simulink model "Motion_planner_Street_Drone"  (R2019b)
settings: Solver=FixedStepAuto  StartTime=0.0  StopTime=25  FixedStep=0.0075  MaxStep=1e-1  MinStep=1e-3  RelTol=1e-3  AbsTol=1e-4
InitFcn:
  | SD_init1
values from neighbouring files (symbols this model uses):
  cost = [2.71432892747 3.32441927977 3.79268757264 4.85642115368 6.12135035287 7.09825974303 9.57278659789 1.55754789407 1.51399555616 2.57723707661 3.8468529147 4.8336387623 ... (2430 elements, 1x2430)]    [matlab.mat]
  Front_brake = [0 2.2085352751 4.15209150797 6.12733711785 8.16604105928 9.79119154879 12.1808659635 14.1242630413 16.1155522836 18.1386900579 20.0839213981 22.1313006548 ... (68 elements, 34x2)]    [Front_brake.mat]
  N = size(X,1)    [curvature.m]
  obsx = [dx1 dx2 dx3 dx4]'    [dynamic_collison.m]    (also in dynamic_detection1.m = [x1 x2 x3 x4]')
  obsy = [dy1 dy2 dy3 dy4]'    [dynamic_collison.m]    (also in dynamic_detection1.m = [y1 y2 y3 y4]')
  x = obs_path(i,1)    [dynamic_collison.m]    (also in dynamic_detection1.m)
  X = [X]    [curvature.m]
  y = obs_path(i,2)    [dynamic_collison.m]    (also in dynamic_detection1.m)
undefined symbols (not defined in the file or in its folder): d, dfin, dini, Ki, Kp, L_0f, lookahead_time, lookahead_time_rev, Rear_brake, sigbuilder_block, steer_ratio, steer_sens, tfin, tini, TPS_0, xfin, Y, yfin, Z
libraries: sm_lib x290, nesl_utility x136, simulink x6, vrlib x2, powerlib_meascontrol x2
(part 3 of 14)

== system Motion_planner_Street_Drone/Trajectory Tracker/KM- StreetDrone/Street_Drone/Vehicle/FL_Suspension ==
  FL Cylinder : sm_lib/Body Elements/Revolved Solid  GraphicAmbientColor=[0.15 0.15 0.15 1.0]  BasedOnType=Mass  CenterOfMass=[0 0 0]  CenterOfMassUnits=m  GraphicDiffuseColor=[0.5 0.5 0.5]  Density=7850  DensityUnits=kg/(m^3)  DoExposeReferenceFrame=off  GraphicEmissiveColor=[0.0 0.0 0.0 1.0]  ExportEntireGeometry=off  SerializedFrames=<Frames><Frame><Id>Frame1</Id><Value><Name>F1</Name><Origin><Source>GeometricFeature</Source><FeatureName>side surface 1</FeatureName></Origin><PrimaryAxis><DefinedDirection>+Z</DefinedDirection><Source>ReferenceFrame</Source><SourceDirection>+Z</SourceDirection><FeatureName></FeatureName></PrimaryAxis><SecondaryAxis><DefinedDirection>+X</DefinedDirection><Source>ReferenceFrame</Source><SourceDirection>+X</SourceDirection><FeatureName></FeatureName></SecondaryAxis></Value></Frame></Frames>  MarkerShape=Sphere  MarkerSize=10  GraphicType=FromGeometry  InertiaType=CalculateFromGeometry  Mass=2  MassUnits=kg  MomentsOfInertia=[1 1 1]  MomentsOfInertiaUnits=kg*m^2  GraphicOpacity=0.6  ProductsOfInertia=[0 0 0]  ProductsOfInertiaUnits=kg*m^2  RevolutionCrossSection=cyl_xsec  RevolutionCrossSectionUnits=cm  RevolutionAngle=180  RevolutionAngleUnits=deg  RevolutionExtent=Full  GraphicShininess=75  GraphicSpecularColor=[0.5 0.5 0.5 1.0]  GraphicVisPropType=SimpleVisualProperties
  FL Piston : sm_lib/Body Elements/Revolved Solid  GraphicAmbientColor=[0.15 0.15 0.15 1.0]  BasedOnType=Mass  CenterOfMass=[0 0 0]  CenterOfMassUnits=m  GraphicDiffuseColor=[0.0 0.4 0.6]  Density=7850  DensityUnits=kg/(m^3)  DoExposeReferenceFrame=off  GraphicEmissiveColor=[0.0 0.0 0.0 1.0]  ExportEntireGeometry=off  SerializedFrames=<Frames><Frame><Id>Frame1</Id><Value><Name>F1</Name><Origin><Source>GeometricFeature</Source><FeatureName>side surface 3</FeatureName></Origin><PrimaryAxis><DefinedDirection>-Z</DefinedDirection><Source>ReferenceFrame</Source><SourceDirection>+Z</SourceDirection><FeatureName></FeatureName></PrimaryAxis><SecondaryAxis><DefinedDirection>+X</DefinedDirection><Source>ReferenceFrame</Source><SourceDirection>+X</SourceDirection><FeatureName></FeatureName></SecondaryAxis></Value></Frame><Frame><Id>Frame2</Id><Value><Name>F2</Name><Origin><Source>GeometricFeature</Source><FeatureName>side surface 1</FeatureName></Origin><PrimaryAxis><DefinedDirection>+Z</DefinedDirection><Source>ReferenceFrame</Source><SourceDirection>+Z</SourceDirection><FeatureName></FeatureName></PrimaryAxis><SecondaryAxis><DefinedDirection>+X</DefinedDirection><Source>ReferenceFrame</Source><SourceDirection>+X</SourceDirection><FeatureName></FeatureName></SecondaryAxis></Value></Frame></Frames>  MarkerShape=Sphere  MarkerSize=10  GraphicType=FromGeometry  InertiaType=CalculateFromGeometry  Mass=2  MassUnits=kg  MomentsOfInertia=[1 1 1]  MomentsOfInertiaUnits=kg*m^2  GraphicOpacity=1.0  ProductsOfInertia=[0 0 0]  ProductsOfInertiaUnits=kg*m^2  RevolutionCrossSection=piston_xsec  RevolutionCrossSectionUnits=cm  RevolutionAngle=180  RevolutionAngleUnits=deg  RevolutionExtent=Full  GraphicShininess=75  GraphicSpecularColor=[0.5 0.5 0.5 1.0]  GraphicVisPropType=SimpleVisualProperties
  PS-Simulink Converter{1..4,20} (5 alike) : nesl_utility/PS-Simulink Converter  PhysicalDomain=network_engine_domain  SubClassName=ps_output  LeftPortType=input  RightPortType=output  PseudoPeriodic=off  Frequencies=[]  Unit=inherit  AffineConversion=off
  Prismatic Joint1 : sm_lib/Joints/Prismatic Joint  JointMode=Normal  SenseConstraintForce=off  SenseConstraintForceX=off  SenseConstraintForceY=off  SenseConstraintForceZ=off  SenseConstraintTorque=off  SenseConstraintTorqueX=off  SenseConstraintTorqueY=off  SenseConstraintTorqueZ=off  SenseTotalForce=off  SenseTotalForceX=off  SenseTotalForceY=off  SenseTotalForceZ=off  SenseTotalTorque=off  SenseTotalTorqueX=off  SenseTotalTorqueY=off  SenseTotalTorqueZ=off  CompositeWrenchDir=FollowerOnBase  CompositeWrenchFrame=BaseFrame  EquilibriumPosition=0.1691  EquilibriumPositionUnits=m  SpringStiffness=50000  SpringStiffnessUnits=N/m  DampingCoefficient=3600  DampingCoefficientUnits=N/(m/s)  TorqueActuationMode=NoTorque  MotionActuationMode=ComputedMotion  SensePosition=on  SenseVelocity=on  SenseAcceleration=off  SenseTorqueForce=on  SenseLowerLimitTorqueForce=on  SenseUpperLimitTorqueForce=on  LowerLimitSpecify=off  LowerLimitBound=0.1  LowerLimitBoundUnits=m  LowerLimitStiffness=60000  LowerLimitStiffnessUnits=N/m  LowerLimitDamping=2000  LowerLimitDampingUnits=N/(m/s)  LowerLimitTransitionRegionWidth=1e-4  LowerLimitTransitionRegionWidthUnits=m  UpperLimitSpecify=off  UpperLimitBound=0.16  UpperLimitBoundUnits=m  UpperLimitStiffness=283333.33  UpperLimitStiffnessUnits=N/m  UpperLimitDamping=2000  UpperLimitDampingUnits=N/(m/s)  UpperLimitTransitionRegionWidth=1e-4  UpperLimitTransitionRegionWidthUnits=m  PositionTargetSpecify=on  PositionTargetPriority=High  PositionTargetValue=0.1691  PositionTargetValueUnits=m  VelocityTargetSpecify=off  VelocityTargetPriority=High  VelocityTargetValue=0  VelocityTargetValueUnits=m/s
  Rigid Transform : sm_lib/Frames and Transforms/Rigid Transform  TranslationMethod=Cartesian  TranslationStandardOffset=0  TranslationLengthUnit=m  TranslationStandardAxis=+Z  TranslationCartesianOffset=[0.90996 0.32189 0.16271]  TranslationROffset=0  TranslationROffsetUnits=m  TranslationZOffset=0  TranslationZOffsetUnits=m  TranslationThetaOffset=0  TranslationThetaOffsetUnits=deg  RotationMethod=None  RotationAngleUnits=deg  RotationStandardAxis=+Z  RotationAngle=0.0  RotationArbitraryAxis=[0 0 1]  FollAlignAxisA=+X  BaseAlignAxisA=+Y  FollAlignAxisB=+Y  BaseAlignAxisB=+Z  RotationSequenceAxes=FollowerAxes  RotationSequence=XYX  RotationSequenceAngles=[0 0 0]  RotationSequenceAnglesUnits=deg  RotationMatrix=[1 0 0; 0 1 0; 0 0 1]
  Rigid Transform2 : sm_lib/Frames and Transforms/Rigid Transform  TranslationMethod=None  TranslationStandardOffset=0  TranslationLengthUnit=m  TranslationStandardAxis=+Z  TranslationCartesianOffset=[0 0 0]  TranslationROffset=0  TranslationROffsetUnits=m  TranslationZOffset=0  TranslationZOffsetUnits=m  TranslationThetaOffset=0  TranslationThetaOffsetUnits=deg  RotationMethod=StandardAxis  RotationAngleUnits=deg  RotationStandardAxis=+Z  RotationAngle=24.85  RotationArbitraryAxis=[0 0 1]  FollAlignAxisA=+X  BaseAlignAxisA=+Y  FollAlignAxisB=+Y  BaseAlignAxisB=+Z  RotationSequenceAxes=FollowerAxes  RotationSequence=XYX  RotationSequenceAngles=[0 0 0]  RotationSequenceAnglesUnits=deg  RotationMatrix=[1 0 0; 0 1 0; 0 0 1]
  Rigid Transform55 : sm_lib/Frames and Transforms/Rigid Transform  TranslationMethod=None  TranslationStandardOffset=0  TranslationLengthUnit=m  TranslationStandardAxis=+Z  TranslationCartesianOffset=[0.90996 0.32189 0.16271]  TranslationROffset=0  TranslationROffsetUnits=m  TranslationZOffset=0  TranslationZOffsetUnits=m  TranslationThetaOffset=0  TranslationThetaOffsetUnits=deg  RotationMethod=StandardAxis  RotationAngleUnits=deg  RotationStandardAxis=+X  RotationAngle=180  RotationArbitraryAxis=[0 0 1]  FollAlignAxisA=+X  BaseAlignAxisA=+Y  FollAlignAxisB=+Y  BaseAlignAxisB=+Z  RotationSequenceAxes=FollowerAxes  RotationSequence=XYX  RotationSequenceAngles=[0 0 0]  RotationSequenceAnglesUnits=deg  RotationMatrix=[1 0 0; 0 1 0; 0 0 1]
  Scope1 : Scope
  Scope2 : Scope
  Scope9 : Scope  NumInputPorts=3
  Spherical Joint : sm_lib/Joints/Spherical Joint  JointMode=Normal  SenseConstraintForce=off  SenseConstraintForceX=off  SenseConstraintForceY=off  SenseConstraintForceZ=off  SenseConstraintTorque=off  SenseConstraintTorqueX=off  SenseConstraintTorqueY=off  SenseConstraintTorqueZ=off  SenseTotalForce=off  SenseTotalForceX=off  SenseTotalForceY=off  SenseTotalForceZ=off  SenseTotalTorque=off  SenseTotalTorqueX=off  SenseTotalTorqueY=off  SenseTotalTorqueZ=off  CompositeWrenchDir=FollowerOnBase  CompositeWrenchFrame=BaseFrame  DefPosRotationMethod=None  DefPosRotationAngleUnits=deg  DefPosRotationStandardAxis=+Z  DefPosRotationAngle=0.0  DefPosRotationArbitraryAxis=[0 0 1]  DefPosFollAlignAxisA=+X  DefPosBaseAlignAxisA=+Y  DefPosFollAlignAxisB=+Y  DefPosBaseAlignAxisB=+Z  DefPosRotationSequenceAxes=FollowerAxes  DefPosRotationSequence=XYX  DefPosRotationSequenceAngles=[0 0 0]  DefPosRotationSequenceAnglesUnits=deg  DefPosRotationMatrix=[1 0 0; 0 1 0; 0 0 1]  EqPosRotationMethod=None  EqPosRotationAngleUnits=deg  EqPosRotationStandardAxis=+Z  EqPosRotationAngle=0.0  EqPosRotationArbitraryAxis=[0 0 1]  EqPosFollAlignAxisA=+X  EqPosBaseAlignAxisA=+Y  EqPosFollAlignAxisB=+Y  EqPosBaseAlignAxisB=+Z  EqPosRotationSequenceAxes=FollowerAxes  EqPosRotationSequence=XYX  EqPosRotationSequenceAngles=[0 0 0]  EqPosRotationSequenceAnglesUnits=deg  EqPosRotationMatrix=[1 0 0; 0 1 0; 0 0 1]  SpringStiffness=0  SpringStiffnessUnits=N*m/deg  DampingCoefficient=0  DampingCoefficientUnits=N*m/(deg/s)  ActuateTorqueX=on  ActuateTorqueY=on  ActuateTorqueZ=on  ActuateTorque=off  TorqueActuationMode=NoTorque  MotionActuationMode=ComputedMotion  ActuationFrame=BaseFrame  SensePosition=off  SenseVelocityX=off  SenseVelocityY=off  SenseVelocityZ=off  SenseVelocity=off  SenseAccelerationX=off  SenseAccelerationY=off  SenseAccelerationZ=off  SenseAcceleration=off  SenseTorqueX=off  SenseTorqueY=off  SenseTorqueZ=off  SenseTorqueForce=off  SenseLowerLimitTorqueMag=off  SenseUpperLimitTorqueMag=off  SensingFrame=BaseFrame  LowerLimitSpecify=off  LowerLimitBound=15  LowerLimitBoundUnits=deg  LowerLimitStiffness=1e4  LowerLimitStiffnessUnits=N*m/deg  LowerLimitDamping=10  LowerLimitDampingUnits=N*m/(deg/s)  LowerLimitTransitionRegionWidth=0.1  LowerLimitTransitionRegionWidthUnits=deg  UpperLimitSpecify=off  UpperLimitBound=45  UpperLimitBoundUnits=deg  UpperLimitStiffness=1e4  UpperLimitStiffnessUnits=N*m/deg  UpperLimitDamping=10  UpperLimitDampingUnits=N*m/(deg/s)  UpperLimitTransitionRegionWidth=0.1  UpperLimitTransitionRegionWidthUnits=deg  PositionTargetRotationMethod=None  PositionTargetRotationAngleUnits=deg  PositionTargetRotationStandardAxis=+Z  PositionTargetRotationAngle=0.0  PositionTargetRotationArbitraryAxis=[0 0 1]  PositionTargetFollAlignAxisA=+X  PositionTargetBaseAlignAxisA=+Y  PositionTargetFollAlignAxisB=+Y  PositionTargetBaseAlignAxisB=+Z  PositionTargetRotationSequenceAxes=FollowerAxes  PositionTargetRotationSequence=XYX  PositionTargetRotationSequenceAngles=[0 0 0]  PositionTargetRotationSequenceAnglesUnits=deg  PositionTargetRotationMatrix=[1 0 0; 0 1 0; 0 0 1]  PositionTargetSpecify=off  PositionTargetPriority=High  VelocityTargetValue=[0 0 0]  VelocityTargetValueUnits=deg/s  VelocityTargetSpecify=off  VelocityTargetPriority=Low  VelocityTargetInFollowerFrame=off
  steering_angle_measurement : Subsystem
  chassis : PMIOPort  Side=Left
  upright : PMIOPort  Port=2  Side=Right
  wires:
  PS-Simulink Converter4/1 -> Scope9/3
  PS-Simulink Converter3/1 -> Scope9/2
  PS-Simulink Converter2/1 -> Scope9/1
  PS-Simulink Converter1/1 -> Scope2/1
  PS-Simulink Converter20/1 -> Scope1/1
  connections:
  Prismatic Joint1/RConn6 -- PS-Simulink Converter4/LConn1
  Prismatic Joint1/RConn5 -- PS-Simulink Converter3/LConn1
  Prismatic Joint1/RConn4 -- PS-Simulink Converter2/LConn1
  Prismatic Joint1/RConn3 -- PS-Simulink Converter1/LConn1
  Rigid Transform2/RConn1 -- upright/RConn1
  Prismatic Joint1/LConn1 -- FL Cylinder/LConn1 -- steering_angle_measurement/RConn1 -- Rigid Transform55/RConn1
  steering_angle_measurement/LConn1 -- chassis/RConn1 -- Rigid Transform/LConn1
  Spherical Joint/LConn1 -- Rigid Transform/RConn1
  Spherical Joint/RConn1 -- Rigid Transform55/LConn1
  FL Piston/RConn1 -- Rigid Transform2/LConn1
  Prismatic Joint1/RConn1 -- FL Piston/LConn1
  Prismatic Joint1/RConn2 -- PS-Simulink Converter20/LConn1

== system Motion_planner_Street_Drone/Trajectory Tracker/KM- StreetDrone/Street_Drone/Vehicle/FL_Upright ==
  Cylindrical Solid1 : sm_lib/Body Elements/Cylindrical Solid  GraphicAmbientColor=[0.15 0.15 0.15 1.0]  BasedOnType=Mass  CenterOfMass=[0 0 0]  CenterOfMassUnits=m  GraphicDiffuseColor=[0.5 0.5 0.5]  CylinderLength=19.061  CylinderLengthUnits=cm  CylinderRadius=1  CylinderRadiusUnits=cm  Density=1000  DensityUnits=kg/m^3  DoExposeReferenceFrame=off  GraphicEmissiveColor=[0.0 0.0 0.0 1.0]  ExportEntireGeometry=off  SerializedFrames=<Frames><Frame><Id>Frame1</Id><Value><Name>F1</Name><Origin><Source>GeometricFeature</Source><FeatureName>top surface</FeatureName></Origin><PrimaryAxis><DefinedDirection>+Z</DefinedDirection><Source>ReferenceFrame</Source><SourceDirection>+Z</SourceDirection><FeatureName></FeatureName></PrimaryAxis><SecondaryAxis><DefinedDirection>+X</DefinedDirection><Source>ReferenceFrame</Source><SourceDirection>+X</SourceDirection><FeatureName></FeatureName></SecondaryAxis></Value></Frame><Frame><Id>Frame2</Id><Value><Name>F2</Name><Origin><Source>GeometricFeature</Source><FeatureName>bottom surface</FeatureName></Origin><PrimaryAxis><DefinedDirection>+Z</DefinedDirection><Source>ReferenceFrame</Source><SourceDirection>+Z</SourceDirection><FeatureName></FeatureName></PrimaryAxis><SecondaryAxis><DefinedDirection>+X</DefinedDirection><Source>ReferenceFrame</Source><SourceDirection>+X</SourceDirection><FeatureName></FeatureName></SecondaryAxis></Value></Frame></Frames>  MarkerShape=Sphere  MarkerSize=10  GraphicType=FromGeometry  InertiaType=CalculateFromGeometry  Mass=3.5  MassUnits=kg  MomentsOfInertia=[0.0001 0.0001 0.0001]  MomentsOfInertiaUnits=kg*m^2  GraphicOpacity=1.0  ProductsOfInertia=[0 0 0]  ProductsOfInertiaUnits=kg*m^2  GraphicShininess=75  GraphicSpecularColor=[0.5 0.5 0.5 1.0]  GraphicVisPropType=SimpleVisualProperties
  Cylindrical Solid10 : sm_lib/Body Elements/Cylindrical Solid  GraphicAmbientColor=[0.15 0.15 0.15 1.0]  BasedOnType=Density  CenterOfMass=[0 0 0]  CenterOfMassUnits=m  GraphicDiffuseColor=[0.5 0.5 0.5]  CylinderLength=4.72  CylinderLengthUnits=cm  CylinderRadius=1  CylinderRadiusUnits=cm  Density=1000  DensityUnits=kg/m^3  DoExposeReferenceFrame=off  GraphicEmissiveColor=[0.0 0.0 0.0 1.0]  ExportEntireGeometry=off  SerializedFrames=<Frames><Frame><Id>Frame1</Id><Value><Name>F1</Name><Origin><Source>GeometricFeature</Source><FeatureName>top surface</FeatureName></Origin><PrimaryAxis><DefinedDirection>+Z</DefinedDirection><Source>ReferenceFrame</Source><SourceDirection>+Z</SourceDirection><FeatureName></FeatureName></PrimaryAxis><SecondaryAxis><DefinedDirection>+X</DefinedDirection><Source>ReferenceFrame</Source><SourceDirection>+X</SourceDirection><FeatureName></FeatureName></SecondaryAxis></Value></Frame><Frame><Id>Frame2</Id><Value><Name>F2</Name><Origin><Source>GeometricFeature</Source><FeatureName>bottom surface</FeatureName></Origin><PrimaryAxis><DefinedDirection>+Z</DefinedDirection><Source>ReferenceFrame</Source><SourceDirection>+Z</SourceDirection><FeatureName></FeatureName></PrimaryAxis><SecondaryAxis><DefinedDirection>+X</DefinedDirection><Source>ReferenceFrame</Source><SourceDirection>+X</SourceDirection><FeatureName></FeatureName></SecondaryAxis></Value></Frame></Frames>  MarkerShape=Sphere  MarkerSize=10  GraphicType=FromGeometry  InertiaType=Custom  Mass=0  MassUnits=kg  MomentsOfInertia=[0 0 0]  MomentsOfInertiaUnits=kg*m^2  GraphicOpacity=1.0  ProductsOfInertia=[0 0 0]  ProductsOfInertiaUnits=kg*m^2  GraphicShininess=75  GraphicSpecularColor=[0.5 0.5 0.5 1.0]  GraphicVisPropType=SimpleVisualProperties
  Cylindrical Solid2 : sm_lib/Body Elements/Cylindrical Solid  GraphicAmbientColor=[0.15 0.15 0.15 1.0]  BasedOnType=Density  CenterOfMass=[0 0 0]  CenterOfMassUnits=m  GraphicDiffuseColor=[0.5 0.5 0.5]  CylinderLength=5  CylinderLengthUnits=cm  CylinderRadius=1  CylinderRadiusUnits=cm  Density=1000  DensityUnits=kg/m^3  DoExposeReferenceFrame=off  GraphicEmissiveColor=[0.0 0.0 0.0 1.0]  ExportEntireGeometry=off  SerializedFrames=<Frames><Frame><Id>Frame1</Id><Value><Name>F1</Name><Origin><Source>GeometricFeature</Source><FeatureName>top surface</FeatureName></Origin><PrimaryAxis><DefinedDirection>+Z</DefinedDirection><Source>ReferenceFrame</Source><SourceDirection>+Z</SourceDirection><FeatureName></FeatureName></PrimaryAxis><SecondaryAxis><DefinedDirection>+X</DefinedDirection><Source>ReferenceFrame</Source><SourceDirection>+X</SourceDirection><FeatureName></FeatureName></SecondaryAxis></Value></Frame><Frame><Id>Frame2</Id><Value><Name>F2</Name><Origin><Source>GeometricFeature</Source><FeatureName>bottom surface</FeatureName></Origin><PrimaryAxis><DefinedDirection>+Z</DefinedDirection><Source>ReferenceFrame</Source><SourceDirection>+Z</SourceDirection><FeatureName></FeatureName></PrimaryAxis><SecondaryAxis><DefinedDirection>+X</DefinedDirection><Source>ReferenceFrame</Source><SourceDirection>+X</SourceDirection><FeatureName></FeatureName></SecondaryAxis></Value></Frame></Frames>  MarkerShape=Sphere  MarkerSize=10  GraphicType=FromGeometry  InertiaType=Custom  Mass=0  MassUnits=kg  MomentsOfInertia=[0 0 0]  MomentsOfInertiaUnits=kg*m^2  GraphicOpacity=1.0  ProductsOfInertia=[0 0 0]  ProductsOfInertiaUnits=kg*m^2  GraphicShininess=75  GraphicSpecularColor=[0.5 0.5 0.5 1.0]  GraphicVisPropType=SimpleVisualProperties
  Cylindrical Solid9 : sm_lib/Body Elements/Cylindrical Solid  GraphicAmbientColor=[0.15 0.15 0.15 1.0]  BasedOnType=Density  CenterOfMass=[0 0 0]  CenterOfMassUnits=m  GraphicDiffuseColor=[0.5 0.5 0.5]  CylinderLength=7.9  CylinderLengthUnits=cm  CylinderRadius=1  CylinderRadiusUnits=cm  Density=1000  DensityUnits=kg/m^3  DoExposeReferenceFrame=off  GraphicEmissiveColor=[0.0 0.0 0.0 1.0]  ExportEntireGeometry=off  SerializedFrames=<Frames><Frame><Id>Frame1</Id><Value><Name>F1</Name><Origin><Source>GeometricFeature</Source><FeatureName>top surface</FeatureName></Origin><PrimaryAxis><DefinedDirection>+Z</DefinedDirection><Source>ReferenceFrame</Source><SourceDirection>+Z</SourceDirection><FeatureName></FeatureName></PrimaryAxis><SecondaryAxis><DefinedDirection>+X</DefinedDirection><Source>ReferenceFrame</Source><SourceDirection>+X</SourceDirection><FeatureName></FeatureName></SecondaryAxis></Value></Frame><Frame><Id>Frame2</Id><Value><Name>F2</Name><Origin><Source>GeometricFeature</Source><FeatureName>bottom surface</FeatureName></Origin><PrimaryAxis><DefinedDirection>+Z</DefinedDirection><Source>ReferenceFrame</Source><SourceDirection>+Z</SourceDirection><FeatureName></FeatureName></PrimaryAxis><SecondaryAxis><DefinedDirection>+X</DefinedDirection><Source>ReferenceFrame</Source><SourceDirection>+X</SourceDirection><FeatureName></FeatureName></SecondaryAxis></Value></Frame></Frames>  MarkerShape=Sphere  MarkerSize=10  GraphicType=FromGeometry  InertiaType=Custom  Mass=0  MassUnits=kg  MomentsOfInertia=[0 0 0]  MomentsOfInertiaUnits=kg*m^2  GraphicOpacity=1.0  ProductsOfInertia=[0 0 0]  ProductsOfInertiaUnits=kg*m^2  GraphicShininess=75  GraphicSpecularColor=[0.5 0.5 0.5 1.0]  GraphicVisPropType=SimpleVisualProperties
  Rigid Transform11 : sm_lib/Frames and Transforms/Rigid Transform  TranslationMethod=StandardAxis  TranslationStandardOffset=9.929  TranslationLengthUnit=cm  TranslationStandardAxis=+Z  TranslationCartesianOffset=[0 0 0]  TranslationROffset=0  TranslationROffsetUnits=m  TranslationZOffset=0  TranslationZOffsetUnits=m  TranslationThetaOffset=0  TranslationThetaOffsetUnits=deg  RotationMethod=StandardAxis  RotationAngleUnits=deg  RotationStandardAxis=+X  RotationAngle=90  RotationArbitraryAxis=[0 0 1]  FollAlignAxisA=+X  BaseAlignAxisA=+Y  FollAlignAxisB=+Y  BaseAlignAxisB=+Z  RotationSequenceAxes=FollowerAxes  RotationSequence=XYX  RotationSequenceAngles=[0 0 0]  RotationSequenceAnglesUnits=deg  RotationMatrix=[1 0 0; 0 1 0; 0 0 1]
  Rigid Transform12 : sm_lib/Frames and Transforms/Rigid Transform  TranslationMethod=StandardAxis  TranslationStandardOffset=0.5  TranslationLengthUnit=cm  TranslationStandardAxis=+Y  TranslationCartesianOffset=[0 0 0]  TranslationROffset=0  TranslationROffsetUnits=m  TranslationZOffset=0  TranslationZOffsetUnits=m  TranslationThetaOffset=0  TranslationThetaOffsetUnits=deg  RotationMethod=StandardAxis  RotationAngleUnits=deg  RotationStandardAxis=-X  RotationAngle=89  RotationArbitraryAxis=[0 0 1]  FollAlignAxisA=+X  BaseAlignAxisA=+Y  FollAlignAxisB=+Y  BaseAlignAxisB=+Z  RotationSequenceAxes=FollowerAxes  RotationSequence=XYX  RotationSequenceAngles=[0 0 0]  RotationSequenceAnglesUnits=deg  RotationMatrix=[1 0 0; 0 1 0; 0 0 1]
  Rigid Transform14 : sm_lib/Frames and Transforms/Rigid Transform  TranslationMethod=StandardAxis  TranslationStandardOffset=0.5  TranslationLengthUnit=cm  TranslationStandardAxis=-Y  TranslationCartesianOffset=[0 0 0]  TranslationROffset=0  TranslationROffsetUnits=m  TranslationZOffset=0  TranslationZOffsetUnits=m  TranslationThetaOffset=0  TranslationThetaOffsetUnits=deg  RotationMethod=StandardAxis  RotationAngleUnits=deg  RotationStandardAxis=-X  RotationAngle=88  RotationArbitraryAxis=[0 0 1]  FollAlignAxisA=+X  BaseAlignAxisA=+Y  FollAlignAxisB=+Y  BaseAlignAxisB=+Z  RotationSequenceAxes=FollowerAxes  RotationSequence=XYX  RotationSequenceAngles=[0 0 0]  RotationSequenceAnglesUnits=deg  RotationMatrix=[1 0 0; 0 1 0; 0 0 1]
  Rigid Transform15 : sm_lib/Frames and Transforms/Rigid Transform  TranslationMethod=None  TranslationStandardOffset=0  TranslationLengthUnit=m  TranslationStandardAxis=+Z  TranslationCartesianOffset=[0 0 0]  TranslationROffset=0  TranslationROffsetUnits=m  TranslationZOffset=0  TranslationZOffsetUnits=m  TranslationThetaOffset=0  TranslationThetaOffsetUnits=deg  RotationMethod=StandardAxis  RotationAngleUnits=deg  RotationStandardAxis=+Y  RotationAngle=180  RotationArbitraryAxis=[0 0 1]  FollAlignAxisA=+X  BaseAlignAxisA=+Y  FollAlignAxisB=+Y  BaseAlignAxisB=+Z  RotationSequenceAxes=FollowerAxes  RotationSequence=XYX  RotationSequenceAngles=[0 0 0]  RotationSequenceAnglesUnits=deg  RotationMatrix=[1 0 0; 0 1 0; 0 0 1]
  Rigid Transform16 : sm_lib/Frames and Transforms/Rigid Transform  TranslationMethod=None  TranslationStandardOffset=9.132  TranslationLengthUnit=cm  TranslationStandardAxis=-Z  TranslationCartesianOffset=[0 0 0]  TranslationROffset=0  TranslationROffsetUnits=m  TranslationZOffset=0  TranslationZOffsetUnits=m  TranslationThetaOffset=0  TranslationThetaOffsetUnits=deg  RotationMethod=StandardAxis  RotationAngleUnits=deg  RotationStandardAxis=+X  RotationAngle=-73  RotationArbitraryAxis=[0 0 1]  FollAlignAxisA=+X  BaseAlignAxisA=+Y  FollAlignAxisB=+Y  BaseAlignAxisB=+Z  RotationSequenceAxes=FollowerAxes  RotationSequence=XYX  RotationSequenceAngles=[0 0 0]  RotationSequenceAnglesUnits=deg  RotationMatrix=[1 0 0; 0 1 0; 0 0 1]
  Rigid Transform17 : sm_lib/Frames and Transforms/Rigid Transform  TranslationMethod=None  TranslationStandardOffset=9.132  TranslationLengthUnit=cm  TranslationStandardAxis=-Z  TranslationCartesianOffset=[0 0 0]  TranslationROffset=0  TranslationROffsetUnits=m  TranslationZOffset=0  TranslationZOffsetUnits=m  TranslationThetaOffset=0  TranslationThetaOffsetUnits=deg  RotationMethod=StandardAxis  RotationAngleUnits=deg  RotationStandardAxis=+X  RotationAngle=-90  RotationArbitraryAxis=[0 0 1]  FollAlignAxisA=+X  BaseAlignAxisA=+Y  FollAlignAxisB=+Y  BaseAlignAxisB=+Z  RotationSequenceAxes=FollowerAxes  RotationSequence=XYX  RotationSequenceAngles=[0 0 0]  RotationSequenceAnglesUnits=deg  RotationMatrix=[1 0 0; 0 1 0; 0 0 1]
  Rigid Transform56 : sm_lib/Frames and Transforms/Rigid Transform  TranslationMethod=StandardAxis  TranslationStandardOffset=9.929  TranslationLengthUnit=cm  TranslationStandardAxis=+Z  TranslationCartesianOffset=[0 0 0]  TranslationROffset=0  TranslationROffsetUnits=m  TranslationZOffset=0  TranslationZOffsetUnits=m  TranslationThetaOffset=0  TranslationThetaOffsetUnits=deg  RotationMethod=StandardAxis  RotationAngleUnits=deg  RotationStandardAxis=-Y  RotationAngle=98.5  RotationArbitraryAxis=[0 0 1]  FollAlignAxisA=+X  BaseAlignAxisA=+Y  FollAlignAxisB=+Y  BaseAlignAxisB=+Z  RotationSequenceAxes=FollowerAxes  RotationSequence=XYX  RotationSequenceAngles=[0 0 0]  RotationSequenceAnglesUnits=deg  RotationMatrix=[1 0 0; 0 1 0; 0 0 1]
  Rigid Transform60 : sm_lib/Frames and Transforms/Rigid Transform  TranslationMethod=None  TranslationStandardOffset=9.929  TranslationLengthUnit=cm  TranslationStandardAxis=+Z  TranslationCartesianOffset=[0 0 0]  TranslationROffset=0  TranslationROffsetUnits=m  TranslationZOffset=0  TranslationZOffsetUnits=m  TranslationThetaOffset=0  TranslationThetaOffsetUnits=deg  RotationMethod=StandardAxis  RotationAngleUnits=deg  RotationStandardAxis=-X  RotationAngle=90  RotationArbitraryAxis=[0 0 1]  FollAlignAxisA=+X  BaseAlignAxisA=+Y  FollAlignAxisB=+Y  BaseAlignAxisB=+Z  RotationSequenceAxes=FollowerAxes  RotationSequence=XYX  RotationSequenceAngles=[0 0 0]  RotationSequenceAnglesUnits=deg  RotationMatrix=[1 0 0; 0 1 0; 0 0 1]
  Rigid Transform61 : sm_lib/Frames and Transforms/Rigid Transform  TranslationMethod=None  TranslationStandardOffset=9.929  TranslationLengthUnit=cm  TranslationStandardAxis=+Z  TranslationCartesianOffset=[0 0 0]  TranslationROffset=0  TranslationROffsetUnits=m  TranslationZOffset=0  TranslationZOffsetUnits=m  TranslationThetaOffset=0  TranslationThetaOffsetUnits=deg  RotationMethod=StandardAxis  RotationAngleUnits=deg  RotationStandardAxis=-Y  RotationAngle=21.3  RotationArbitraryAxis=[0 0 1]  FollAlignAxisA=+X  BaseAlignAxisA=+Y  FollAlignAxisB=+Y  BaseAlignAxisB=+Z  RotationSequenceAxes=FollowerAxes  RotationSequence=XYX  RotationSequenceAngles=[0 0 0]  RotationSequenceAnglesUnits=deg  RotationMatrix=[1 0 0; 0 1 0; 0 0 1]
  upright1 : sm_lib/Body Elements/Brick Solid  GraphicAmbientColor=[0.15 0.15 0.15 1.0]  BasedOnType=Density  BrickDimensions=[1 1 9.265]  BrickDimensionUnits=cm  CenterOfMass=[0 0 0]  CenterOfMassUnits=m  GraphicDiffuseColor=[0.5 0.5 0.5]  Density=1000  DensityUnits=kg/m^3  DoExposeReferenceFrame=off  GraphicEmissiveColor=[0.0 0.0 0.0 1.0]  ExportEntireGeometry=off  SerializedFrames=<Frames><Frame><Id>Frame1</Id><Value><Name>F1</Name><Origin><Source>GeometricFeature</Source><FeatureName>+y +z curve</FeatureName></Origin><PrimaryAxis><DefinedDirection>+Z</DefinedDirection><Source>ReferenceFrame</Source><SourceDirection>+Z</SourceDirection><FeatureName></FeatureName></PrimaryAxis><SecondaryAxis><DefinedDirection>+X</DefinedDirection><Source>ReferenceFrame</Source><SourceDirection>+X</SourceDirection><FeatureName></FeatureName></SecondaryAxis></Value></Frame><Frame><Id>Frame2</Id><Value><Name>F2</Name><Origin><Source>GeometricFeature</Source><FeatureName>-z surface</FeatureName></Origin><PrimaryAxis><DefinedDirection>+Z</DefinedDirection><Source>ReferenceFrame</Source><SourceDirection>+Z</SourceDirection><FeatureName></FeatureName></PrimaryAxis><SecondaryAxis><DefinedDirection>+X</DefinedDirection><Source>ReferenceFrame</Source><SourceDirection>+X</SourceDirection><FeatureName></FeatureName></SecondaryAxis></Value></Frame></Frames>  MarkerShape=Sphere  MarkerSize=10  GraphicType=FromGeometry  InertiaType=Custom  Mass=0  MassUnits=kg  MomentsOfInertia=[0 0 0]  MomentsOfInertiaUnits=kg*m^2  GraphicOpacity=0.75  ProductsOfInertia=[0 0 0]  ProductsOfInertiaUnits=kg*m^2  GraphicShininess=75  GraphicSpecularColor=[0.5 0.5 0.5 1.0]  GraphicVisPropType=SimpleVisualProperties
  upright2 : sm_lib/Body Elements/Brick Solid  GraphicAmbientColor=[0.15 0.15 0.15 1.0]  BasedOnType=Density  BrickDimensions=[1 1 3.5]  BrickDimensionUnits=cm  CenterOfMass=[0 0 0]  CenterOfMassUnits=m  GraphicDiffuseColor=[0.5 0.5 0.5]  Density=1000  DensityUnits=kg/m^3  DoExposeReferenceFrame=off  GraphicEmissiveColor=[0.0 0.0 0.0 1.0]  ExportEntireGeometry=off  SerializedFrames=<Frames><Frame><Id>Frame1</Id><Value><Name>F1</Name><Origin><Source>GeometricFeature</Source><FeatureName>-y +z curve</FeatureName></Origin><PrimaryAxis><DefinedDirection>+Z</DefinedDirection><Source>ReferenceFrame</Source><SourceDirection>+Z</SourceDirection><FeatureName></FeatureName></PrimaryAxis><SecondaryAxis><DefinedDirection>+X</DefinedDirection><Source>ReferenceFrame</Source><SourceDirection>+X</SourceDirection><FeatureName></FeatureName></SecondaryAxis></Value></Frame><Frame><Id>Frame2</Id><Value><Name>F2</Name><Origin><Source>GeometricFeature</Source><FeatureName>-z surface</FeatureName></Origin><PrimaryAxis><DefinedDirection>+Z</DefinedDirection><Source>ReferenceFrame</Source><SourceDirection>+Z</SourceDirection><FeatureName></FeatureName></PrimaryAxis><SecondaryAxis><DefinedDirection>+X</DefinedDirection><Source>ReferenceFrame</Source><SourceDirection>+X</SourceDirection><FeatureName></FeatureName></SecondaryAxis></Value></Frame></Frames>  MarkerShape=Sphere  MarkerSize=10  GraphicType=FromGeometry  InertiaType=Custom  Mass=0  MassUnits=kg  MomentsOfInertia=[0 0 0]  MomentsOfInertiaUnits=kg*m^2  GraphicOpacity=0.75  ProductsOfInertia=[0 0 0]  ProductsOfInertiaUnits=kg*m^2  GraphicShininess=75  GraphicSpecularColor=[0.5 0.5 0.5 1.0]  GraphicVisPropType=SimpleVisualProperties
  arm : PMIOPort  Side=Left
  wheel : PMIOPort  Port=2  Side=Right
  steering_rack : PMIOPort  Port=3  Side=Left
  suspension : PMIOPort  Port=4  Side=Left
  connections:
  Rigid Transform17/RConn1 -- arm/RConn1
  steering_rack/RConn1 -- Cylindrical Solid10/RConn1
  Rigid Transform12/LConn1 -- upright1/RConn1
  Cylindrical Solid1/RConn1 -- Rigid Transform14/RConn1 -- Rigid Transform56/LConn1 -- Rigid Transform11/LConn1
  Rigid Transform60/LConn1 -- Cylindrical Solid9/RConn1
  Rigid Transform15/LConn1 -- Cylindrical Solid2/RConn1
  suspension/RConn1 -- Rigid Transform16/RConn1
  Rigid Transform17/LConn1 -- upright2/LConn1
  Cylindrical Solid9/LConn1 -- Rigid Transform56/RConn1
  Rigid Transform12/RConn1 -- Cylindrical Solid1/LConn1
  upright2/RConn1 -- Rigid Transform14/LConn1
  wheel/RConn1 -- Rigid Transform15/RConn1
  Cylindrical Solid2/LConn1 -- Rigid Transform11/RConn1
  Rigid Transform61/LConn1 -- Rigid Transform60/RConn1
  Rigid Transform16/LConn1 -- upright1/LConn1
  Cylindrical Solid10/LConn1 -- Rigid Transform61/RConn1

== system Motion_planner_Street_Drone/Trajectory Tracker/KM- StreetDrone/Street_Drone/Vehicle/FL_Wheel ==
  For Validation : Subsystem
  Non-moving road : Subsystem  mask{dummy=off}
  Scaling factors : Subsystem  Tag=Scaling factors  mask{LMUX=1, LKX=1, LMUY=1, LKY=1, LKYC=1, LTR=1, LKZC=1}
      mask prompts: LMUX "longitudinal friction"; LKX "longitudinal slip stiffness"; LMUY "lateral fiction"; LKY "cornering stiffness"; LKYC "camber stiffness"; LTR "pneumatic trail"; LKZC "camber torque stiffness"
  Scope : Scope
  SimMechanics2G Wheel + tyre : Subsystem  Tag=SimMechanics Wheel + tyre  mask(SimMechanics_tyre){idtyre=1, inertia=[4.7 0.0593 0.0911], tpfname='SD_car_125_80R13', rdfname='TNO_FlatRoad.rdf', side_mode=(1xxx) left, cnt_mode=(x1xx) smooth road, dyn_mode=(xx2x) relaxation behaviour - non-linear, mf_mode=(xxx3) uncombined, use_mode=1e8, disp_debug=off}
      mask prompts: idtyre "Tyre ID [integer]"; inertia "Rim inertia [3x real] mass (kg) Ixx Iyy (kgm2)"; tpfname "Tyre properties [string or struct]"; rdfname "Road data file [string]"; side_mode "Tyre side            :"; cnt_mode "Contact method :"; dyn_mode "Dynamics           :"; mf_mode "Slip forces          :"; use_mode "Optional: use mode (overrides pop-up) [current selection: 1123]"; disp_debug "Display debug messages"
      mask help:
      | Wheel + tyre model to be used in combination with the SimMechanics multibody toolbox.
      |
      | Tyre model version: MF-Tyre/MF-Swift 6.2
      | © 1996-2013 TNO, Helmond, The Netherlands
      mask init:
      | % initialize parameters
      | % (required to overcome a bug in MATLAB 2006a: errors in a mask are not displayed,
      | %  and simulation is not ended. This check is carried out in s-function 
      | %  'chech_inertia_parameters' in the subsystem)
      | radius     = 1;
      | width      = 1;
      | belt_mass  = 1;
      | belt_Ixx   = 1;
      | belt_Iyy   = 1;
      | tyre_mass  = 1;
      | tyre_Ixx   = 1;
      | tyre_Iyy   = 1;
      | mass = 1;
      | Imat = [1 0 0; 0 1 0; 0 0 1];
      | 
      | % switch between tpf file or struct
      | if ischar(tpfname)
      |     typarr=zeros(300,1);
      |     tpfname_dummy=tpfname;
      |     if ~exist(tpfname_dummy)
      |         error('Tyre property file does not exist')
      |     end
      | elseif isstruct(tpfname)
      |     typarr=tno_tpf_struct2array(tpfname,idtyre);
      |     tpfname_dummy='';
      | else
      |     typarr=zeros(300,1);
      |     tpfname_dummy='';
      |     error(['Mask parameter ''Tyre property file'' should be supplied as string or structure for tyre ' num2str(idtyre)])
      | end
      | if ~exist(rdfname) && ~strcmp(rdfname,'')
      |     error('Road data file does not exist')
      | end
      | 
      | %initialisation script for SimMechanics
      | idroad=1;
      | 
      | %rim inertia as specified by the user in the GUI
      | rim_mass = inertia(1);
      | rim_Ixx  = inertia(2);
      | rim_Iyy  = inertia(3);
      | 
      | % check the use_mode of the model
      | if (abs(use_mode) > 4535 )
      |   iswtch=1000*side_mode+100*cnt_mode+10*(dyn_mode-1)+(mf_mode-1);
      | else
      |   iswtch=use_mode;
      | end
      | 
      | %get tyre inertia parameters from the tyre property file
      | if ischar(tpfname)
      |     [x,typarr]=dteval(tpfname_dummy,[1 2 3 4 5 6],1);
      | end
      | radius     = typarr(7);
      | width      = typarr(8);
      | belt_mass  = typarr(164);
      | belt_Ixx   = typarr(195);
      | belt_Iyy   = typarr(162);
      | tyre_mass  = typarr(190);
      | tyre_Ixx   = typarr(191);
      | tyre_Iyy   = typarr(192);
      | 
      | % display the use_mode of the model
      | if (disp_debug) disp(['Delft-Tyre ' num2str(idtyre) ' -> use_mode=' num2str(iswtch) ]); end
      | 
      | % check and calculate inertia of the rim_body
      | if  ( rim_mass <= 0 | rim_Ixx <= 0 | rim_Iyy <= 0 | tyre_mass <= 0 | tyre_Ixx <= 0 | tyre_Iyy <= 0 | belt_mass <= 0 | belt_Ixx <= 0 | belt_Iyy <= 0 )
      |   error('initialisation calculation results in a negative mass and/or inertia!') 
      |   disp_debug=1;
      | end
      | if  ( tyre_mass <= belt_mass | tyre_Ixx <= belt_Ixx | tyre_Iyy <= belt_Iyy  )
      |   error('initialisation calculation error: tyre belt mass/inertia > tyre mass/inertia!') 
      |   disp_debug=1;
      | end
      | 
      | if (disp_debug) 
      |   msg=[' wheel mass = ',num2str(rim_mass+tyre_mass),' kg'];
      |   disp(msg);
      |   msg=[' wheel Ixx  = ',num2str(rim_Ixx+tyre_Ixx),' kgm2'];
      |   disp(msg);
      |   msg=[' wheel Iyy  = ',num2str(rim_Iyy+tyre_Iyy),' kgm2'];
      |   disp(msg);
      |   msg=[' tyre mass  = ',num2str(tyre_mass),' kg (belt mass = ',num2str(belt_mass),' kg)' ];
      |   disp(msg);
      |   msg=[' tyre Ixx   = ',num2str(tyre_Ixx) ,' kgm2 (belt Ixx  = ',num2str(belt_Ixx) ,' kgm2)'];
      |   disp(msg);
      |   msg=[' tyre Iyy   = ',num2str(tyre_Iyy) ,' kgm2 (belt Iyy  = ',num2str(belt_Iyy) ,' kgm2)'];
      |   disp(msg);
      | end
      | 
      | % calculate the mass of the wheelbody in the MBS environment 
      | %   normally           : rim + tyre
      | %   rigid ring dynamics: rim + part of tyre (and separate rigid body inside tyre model)
      | dynmod=iswtch-100*floor(iswtch/100);
      | if (dynmod/10 >= 3) 
      |   %rigid ring dynamics switched on
      |   wheelbody_mass = rim_mass + tyre_mass - belt_mass;
      |   wheelbody_Ixx  = rim_Ixx  + tyre_Ixx  - belt_Ixx;
      |   wheelbody_Iyy  = rim_Iyy  + tyre_Iyy  - belt_Iyy;
      | else
      |   %rigid ring dynamics switched off
      |   wheelbody_mass = rim_mass + tyre_mass;
      |   wheelbody_Ixx  = rim_Ixx  + tyre_Ixx;
      |   wheelbody_Iyy  = rim_Iyy  + tyre_Iyy;
      | end
      | 
      | mass = wheelbody_mass;
      | Imat = [wheelbody_Ixx 0 0; 0 wheelbody_Iyy 0; 0 0 wheelbody_Ixx]; 
      | 
      | fliplr = 0;
      | % CHANGE GEOMETRY ORIENTATION IF WHEEL IS ON RIGHT SIDE
      | if (side_mode == 2)
      |     fliplr=1;
      |     %disp(['Tyre ID = ' num2str(idtyre) ', fliplr = ' num2str(fliplr)]);
      | end
      mask Help: eval('DTOpenHelp(507)')
      mask TypeOptions side_mode: (1xxx) left | (2xxx) right | (3xxx) symmetric
      mask Callback side_mode:
      | promtstr = get_param(gcb,'MaskPromptString');
      | index = find(double(promtstr)==124);
      | maskval = get_param(gcb,'MaskValues');
      | new_mode = [maskval{5}(2) maskval{6}(3) maskval{7}(4) maskval{8}(5)];
      | newpromtstr = [promtstr(1:index(8)) ['Optional: use mode (overrides pop-up) [current selection: ' new_mode ']'] promtstr(index(9):end)];
      | set_param(gcb,'MaskPromptString',newpromtstr);
      mask TypeOptions cnt_mode: (x1xx) smooth road | (x2xx) smooth road (motorcycle: circular cross section) | (x3xx) moving road | (x4xx) 2D short wavelength road contact | (x5xx) 3D short wavelength road contact
      mask Callback cnt_mode:
      | promtstr = get_param(gcb,'MaskPromptString');
      | index = find(double(promtstr)==124);
      | maskval = get_param(gcb,'MaskValues');
      | new_mode = [maskval{5}(2) maskval{6}(3) maskval{7}(4) maskval{8}(5)];
      | newpromtstr = [promtstr(1:index(8)) ['Optional: use mode (overrides pop-up) [current selection: ' new_mode ']'] promtstr(index(9):end)];
      | set_param(gcb,'MaskPromptString',newpromtstr);
      mask TypeOptions dyn_mode: (xx0x) steady-state | (xx1x) relaxation behaviour | (xx2x) relaxation behaviour - non-linear | (xx3x) rigid ring | (xx4x) rigid ring + initial statics
      mask Callback dyn_mode:
      | promtstr = get_param(gcb,'MaskPromptString');
      | index = find(double(promtstr)==124);
      | maskval = get_param(gcb,'MaskValues');
      | new_mode = [maskval{5}(2) maskval{6}(3) maskval{7}(4) maskval{8}(5)];
      | newpromtstr = [promtstr(1:index(8)) ['Optional: use mode (overrides pop-up) [current selection: ' new_mode ']'] promtstr(index(9):end)];
      | set_param(gcb,'MaskPromptString',newpromtstr);
      mask TypeOptions mf_mode: (xxx0) none | (xxx1) longitudinal | (xxx2) lateral | (xxx3) uncombined | (xxx4) combined | (xxx5) combined+turnslip
      mask Callback mf_mode:
      | promtstr = get_param(gcb,'MaskPromptString');
      | index = find(double(promtstr)==124);
      | maskval = get_param(gcb,'MaskValues');
      | new_mode = [maskval{5}(2) maskval{6}(3) maskval{7}(4) maskval{8}(5)];
      | newpromtstr = [promtstr(1:index(8)) ['Optional: use mode (overrides pop-up) [current selection: ' new_mode ']'] promtstr(index(9):end)];
      | set_param(gcb,'MaskPromptString',newpromtstr);
  Terminator : Terminator
  To Workspace : ToWorkspace  VariableName=varinf1  SampleTime=-1
  r_joint : PMIOPort  Side=Left
  wires:
  SimMechanics2G Wheel + tyre/1(varinf) -> To Workspace/1, Scope/1, For Validation/1(Inputs)
  SimMechanics2G Wheel + tyre/2(body sensor) -> Terminator/1
  Scaling factors/1(scaling) -> SimMechanics2G Wheel + tyre/2(scaling)
  Non-moving road/1(road) -> SimMechanics2G Wheel + tyre/1(road)
  connections:
  SimMechanics2G Wheel + tyre/LConn1 -- r_joint/RConn1
